simulink model "just_the_dynamics"  (R2017b)
settings: Solver=ode45  StartTime=0.0  StopTime=5000  RelTol=1e-3  EnableMultiTasking=on
undefined symbols (not defined in the file): a1, a2, a3, a4, b1, b2, b3, b4, c, c_mi_x, c_mi_y, c_mi_z, co_x, co_y, co_z, d, d_omega_R10, d_omega_R20, d_omega_R30, d_omega_R40, dfi_0, dpsi_0, dtheta_0, dx_0, dy_0, dz_0, f, fi_0, g, ga, h, Ixx, Iyy, Izz, Jr, K, L, m, psi_0, stateref, Tau, theta_0, V1_WP, V2_WP, V3_WP, V4_WP, x_0, y_0, z_0
settings Model: Creator=Jake  LastModifiedBy=Padraig Lysandrou
settings DataIOCC: LimitDataPoints=on  SaveFormat=Array  SignalLoggingSaveFormat=ModelDataLogs
settings OptimizationCC: InitFltsAndDblsToZero=on  LifeSpan=inf
settings DebuggingCC: SaveWithParameterizedLinksMsg=none  UnderspecifiedInitializationDetection=Classic  MergeDetectMultiDrivingBlocksExec=none  SignalResolutionControl=TryResolveAllWithWarning  SolverPrmCheckMsg=warning  MultiTaskDSMMsg=warning  MultiTaskCondExecSysMsg=none  FcnCallInpInsideContextMsg=warning  StrictBusMsg=Warning  SFUnexpectedBacktrackingDiag=warning  SFNoUnconditionalDefaultTransitionDiag=warning  SFExecutionAtInitializationDiag=none
settings HardwareCC: ProdBitPerPointer=32  ProdBitPerSizeT=32  ProdBitPerPtrDiffT=32  ProdLargestAtomicFloat=None  ProdIntDivRoundTo=Undefined  ProdEndianess=Unspecified  ProdWordSize=32  ProdHWDeviceType=32-bit Generic
settings ModelReferenceCC: PropagateSignalLabelsOutOfModel=off
settings SFSimCC: SimParseCustomCode=off
settings CodeAppCC: StateflowObjectComments=on
settings GRTTargetCC: TargetFcnLib=ansi_tfl_tmw.mat  TargetLangStandard=C89/C90 (ANSI)  CombineOutputUpdateFcns=off  GRTInterface=on
settings ConfigComp: CovMetricSettings=dw  CovHtmlReporting=on  CovSaveCumulativeToWorkspaceVar=on  CovSaveSingleToWorkspaceVar=on  CovExternalEMLEnable=off

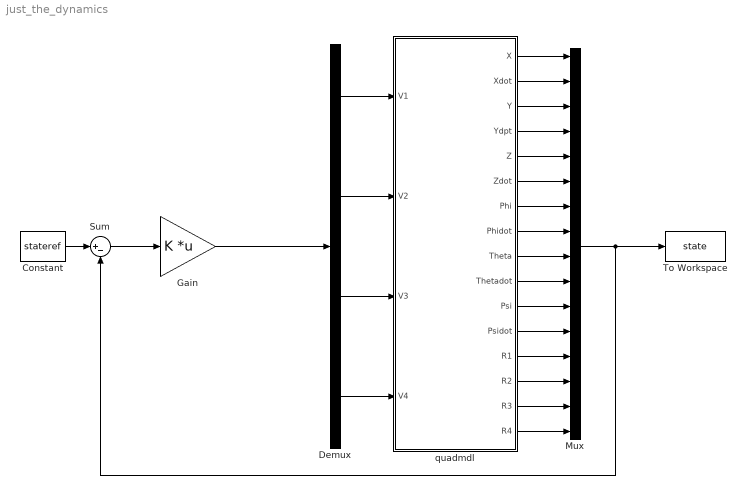
== system just_the_dynamics ==
  Constant : Constant  Value=stateref
  Demux : Demux
  Gain : Gain  Gain=K  Multiplication=Matrix(K*u) (u vector)
  Mux : Mux  Inputs=16
  Sum : Sum  Inputs=|+-
  To Workspace : ToWorkspace  VariableName=state  SaveFormat=Timeseries  SampleTime=-1
  quadmdl : Subsystem
  wires:
  quadmdl/1(X) -> Mux/1
  quadmdl/2(Xdot) -> Mux/2
  quadmdl/3(Y) -> Mux/3
  quadmdl/4(Ydpt) -> Mux/4
  quadmdl/5(Z) -> Mux/5
  quadmdl/6(Zdot) -> Mux/6
  quadmdl/7(Phi) -> Mux/7
  quadmdl/8(Phidot) -> Mux/8
  quadmdl/9(Theta) -> Mux/9
  quadmdl/10(Thetadot) -> Mux/10
  quadmdl/11(Psi) -> Mux/11
  quadmdl/12(Psidot) -> Mux/12
  quadmdl/13(R1) -> Mux/13
  quadmdl/14(R2) -> Mux/14
  quadmdl/15(R3) -> Mux/15
  quadmdl/16(R4) -> Mux/16
  Demux/1 -> quadmdl/1(V1)
  Demux/2 -> quadmdl/2(V2)
  Demux/3 -> quadmdl/3(V3)
  Demux/4 -> quadmdl/4(V4)
  Mux/1 -> Sum/2, To Workspace/1
  Gain/1 -> Demux/1
  Sum/1 -> Gain/1
  Constant/1 -> Sum/1

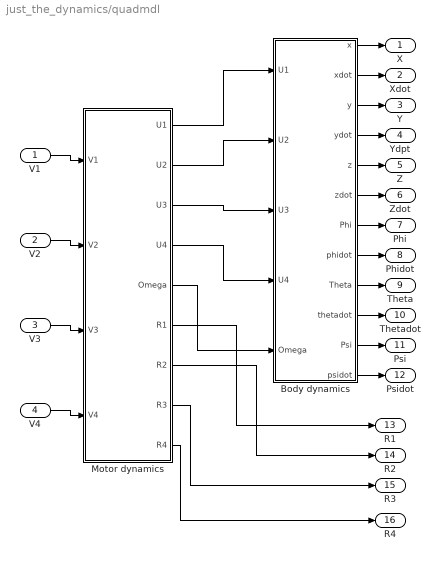
== system just_the_dynamics/quadmdl ==
  V1 : Inport
  V2 : Inport  Port=2
  V3 : Inport  Port=3
  V4 : Inport  Port=4
  Body dynamics : Subsystem
  Motor dynamics : Subsystem
  X : Outport
  Xdot : Outport  Port=2
  Y : Outport  Port=3
  Ydpt : Outport  Port=4
  Z : Outport  Port=5
  Zdot : Outport  Port=6
  Phi : Outport  Port=7
  Phidot : Outport  Port=8
  Theta : Outport  Port=9
  Thetadot : Outport  Port=10
  Psi : Outport  Port=11
  Psidot : Outport  Port=12
  R1 : Outport  Port=13
  R2 : Outport  Port=14
  R3 : Outport  Port=15
  R4 : Outport  Port=16
  wires:
  Motor dynamics/1(U1) -> Body dynamics/1(U1)
  Motor dynamics/2(U2) -> Body dynamics/2(U2)
  Motor dynamics/3(U3) -> Body dynamics/3(U3)
  Motor dynamics/4(U4) -> Body dynamics/4(U4)
  Motor dynamics/5(Omega) -> Body dynamics/5(Omega)
  Body dynamics/7(Phi) -> Phi/1
  Body dynamics/9(Theta) -> Theta/1
  Body dynamics/11(Psi) -> Psi/1
  Body dynamics/1(x) -> X/1
  V1/1 -> Motor dynamics/1(V1)
  Body dynamics/3(y) -> Y/1
  V2/1 -> Motor dynamics/2(V2)
  Body dynamics/5(z) -> Z/1
  V3/1 -> Motor dynamics/3(V3)
  V4/1 -> Motor dynamics/4(V4)
  Body dynamics/2(xdot) -> Xdot/1
  Body dynamics/4(ydot) -> Ydpt/1
  Body dynamics/6(zdot) -> Zdot/1
  Body dynamics/8(phidot) -> Phidot/1
  Body dynamics/10(thetadot) -> Thetadot/1
  Body dynamics/12(psidot) -> Psidot/1
  Motor dynamics/6(R1) -> R1/1
  Motor dynamics/7(R2) -> R2/1
  Motor dynamics/8(R3) -> R3/1
  Motor dynamics/9(R4) -> R4/1

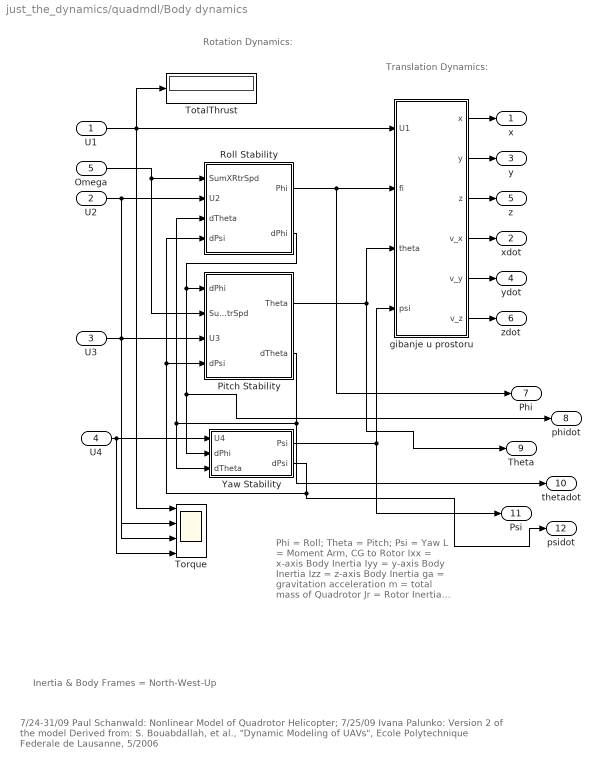
== system just_the_dynamics/quadmdl/Body dynamics ==
  note: Inertia & Body Frames = North-West-Up
  note: Rotation
      | Dynamics:
  note: Translation
      | Dynamics:
  note: Phi = Roll; Theta = Pitch; Psi = Yaw
      | L = Moment Arm, CG to Rotor
      | Ixx = x-axis Body Inertia
      | Iyy = y-axis Body Inertia
      | Izz = z-axis Body Inertia
      | ga = gravitation acceleration
      | m = total mass of Quadrotor
      | Jr = Rotor Inertia
      | a,b = Volts-to-Rotor Speed Consts
      | c,d,e = RtrSpd-to-Thrust Fcn Consts
      | f,g,h = RtrSpd-to-Drag Fcn Consts
      | Tau = Motor Time Const
  note: 7/24-31/09  Paul Schanwald:  Nonlinear Model of Quadrotor Helicopter; 7/25/09 Ivana Palunko: Version 2 of the model
      | Derived from: S. Bouabdallah, et al., "Dynamic Modeling of UAVs", Ecole Polytechnique Federale de Lausanne, 5/2006
  U1 : Inport
  U2 : Inport  Port=2
  U3 : Inport  Port=3
  U4 : Inport  Port=4
  Omega : Inport  Port=5
  Pitch Stability : Subsystem
  Roll Stability : Subsystem
  Torque : Scope  NumInputPorts=4
  TotalThrust : Display
  Yaw Stability : Subsystem
  gibanje u prostoru : Subsystem
  x : Outport
  xdot : Outport  Port=2
  y : Outport  Port=3
  ydot : Outport  Port=4
  z : Outport  Port=5
  zdot : Outport  Port=6
  Phi : Outport  Port=7
  phidot : Outport  Port=8
  Theta : Outport  Port=9
  thetadot : Outport  Port=10
  Psi : Outport  Port=11
  psidot : Outport  Port=12
  wires:
  U4/1 -> Yaw Stability/1(U4), Torque/4
  U3/1 -> Pitch Stability/3(U3), Torque/3
  U1/1 -> TotalThrust/1, gibanje u prostoru/1(U1), Torque/1
  gibanje u prostoru/3(z) -> z/1
  gibanje u prostoru/2(y) -> y/1
  gibanje u prostoru/1(x) -> x/1
  U2/1 -> Roll Stability/2(U2), Torque/2
  Omega/1 -> Roll Stability/1(SumXRtrSpd), Pitch Stability/2(SumYRtrSpd)
  Roll Stability/2(dPhi) -> Pitch Stability/1(dPhi), phidot/1, Yaw Stability/2(dPhi)
  Pitch Stability/2(dTheta) -> thetadot/1, Yaw Stability/3(dTheta), Roll Stability/3(dTheta)
  Yaw Stability/2(dPsi) -> psidot/1, Roll Stability/4(dPsi), Pitch Stability/4(dPsi)
  Roll Stability/1(Phi) -> gibanje u prostoru/2(fi), Phi/1
  Pitch Stability/1(Theta) -> gibanje u prostoru/3(theta), Theta/1
  Yaw Stability/1(Psi) -> Psi/1, gibanje u prostoru/4(psi)
  gibanje u prostoru/6(v_z) -> zdot/1
  gibanje u prostoru/4(v_x) -> xdot/1
  gibanje u prostoru/5(v_y) -> ydot/1

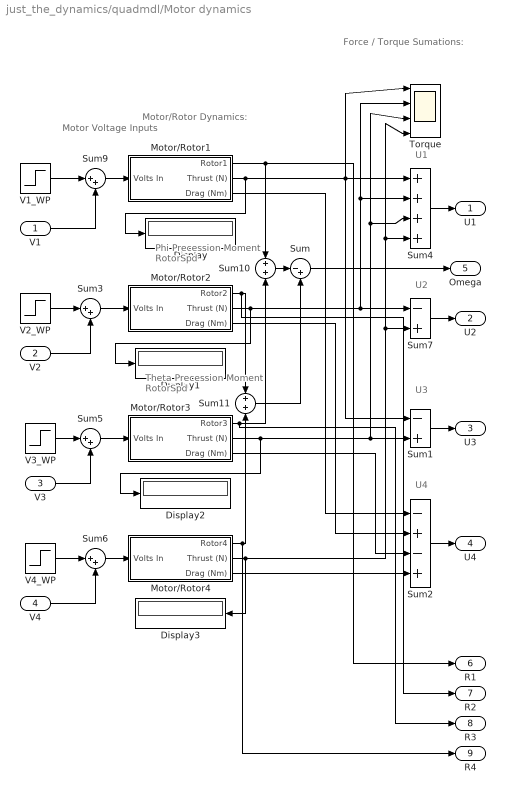
== system just_the_dynamics/quadmdl/Motor dynamics ==
  note: Theta Precession
      | Moment RotorSpd
  note: Phi Precession
      | Moment RotorSpd
  note: Motor/Rotor
      | Dynamics:
  note: Force / Torque
      | Sumations:
  note: Motor
      | Voltage
      | Inputs
  note: U4
  note: U3
  note: U2
  note: U1
  V1 : Inport
  V2 : Inport  Port=2
  V3 : Inport  Port=3
  V4 : Inport  Port=4
  Display{,1..3} (4 alike) : Display
  Motor/Rotor1 : Subsystem
  Motor/Rotor2 : Subsystem
  Motor/Rotor3 : Subsystem
  Motor/Rotor4 : Subsystem
  Sum : Sum  Inputs=|-+
  Sum1 : Sum  Inputs=-+
  Sum10 : Sum  Inputs=+|+
  Sum11 : Sum  Inputs=+|+
  Sum2 : Sum  Inputs=-+-+
  Sum{3,5..6,9} (4 alike) : Sum  Inputs=|++
  Sum4 : Sum  Inputs=++++
  Sum7 : Sum  Inputs=-+
  Torque : Scope  NumInputPorts=4
  V1_WP : Step  Time=0  Before=V1_WP  After=V1_WP  SampleTime=0
  V2_WP : Step  Time=0  Before=V2_WP  After=V2_WP  SampleTime=0
  V3_WP : Step  Time=0  Before=V3_WP  After=V3_WP  SampleTime=0
  V4_WP : Step  Time=0  Before=V4_WP  After=V4_WP  SampleTime=0
  U1 : Outport
  U2 : Outport  Port=2
  U3 : Outport  Port=3
  U4 : Outport  Port=4
  Omega : Outport  Port=5
  R1 : Outport  Port=6
  R2 : Outport  Port=7
  R3 : Outport  Port=8
  R4 : Outport  Port=9
  wires:
  Sum11/1 -> Sum/2
  Sum10/1 -> Sum/1
  Motor/Rotor4/1(Rotor4) -> R4/1, Sum11/2
  Motor/Rotor4/2(Thrust (N)) -> Display3/1, Torque/4, Sum4/4, Sum7/2
  Motor/Rotor4/3(Drag (Nm)) -> Sum2/4
  Motor/Rotor3/3(Drag (Nm)) -> Sum2/3
  Motor/Rotor3/1(Rotor3) -> R3/1, Sum10/2
  Motor/Rotor3/2(Thrust (N)) -> Display2/1, Torque/3, Sum4/3, Sum1/2
  Motor/Rotor2/1(Rotor2) -> R2/1, Sum11/1
  Motor/Rotor2/3(Drag (Nm)) -> Sum2/2
  Motor/Rotor2/2(Thrust (N)) -> Display1/1, Torque/2, Sum4/2, Sum7/1
  Motor/Rotor1/1(Rotor1) -> R1/1, Sum10/1
  Motor/Rotor1/3(Drag (Nm)) -> Sum2/1
  Motor/Rotor1/2(Thrust (N)) -> Display/1, Sum4/1, Torque/1, Sum1/1
  Sum4/1 -> U1/1
  Sum/1 -> Omega/1
  Sum7/1 -> U2/1
  Sum1/1 -> U3/1
  Sum2/1 -> U4/1
  Sum9/1 -> Motor/Rotor1/1(Volts In)
  V1_WP/1 -> Sum9/1
  V2_WP/1 -> Sum3/1
  Sum3/1 -> Motor/Rotor2/1(Volts In)
  V3_WP/1 -> Sum5/1
  Sum5/1 -> Motor/Rotor3/1(Volts In)
  V4_WP/1 -> Sum6/1
  Sum6/1 -> Motor/Rotor4/1(Volts In)
  V1/1 -> Sum9/2
  V2/1 -> Sum3/2
  V3/1 -> Sum5/2
  V4/1 -> Sum6/2

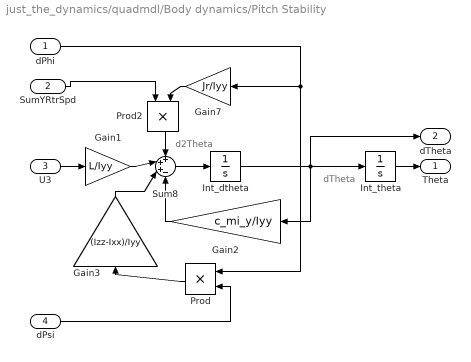
== system just_the_dynamics/quadmdl/Body dynamics/Pitch Stability ==
  note: d2Theta
  note: dTheta
  dPhi : Inport
  SumYRtrSpd : Inport  Port=2
  U3 : Inport  Port=3
  dPsi : Inport  Port=4
  Gain1 : Gain  Gain=L/Iyy
  Gain2 : Gain  Gain=c_mi_y/Iyy
  Gain3 : Gain  Gain=(Izz-Ixx)/Iyy
  Gain7 : Gain  Gain=Jr/Iyy
  Int_dtheta : Integrator  InitialCondition=dtheta_0
  Int_theta : Integrator  InitialCondition=theta_0  UpperSaturationLimit=pi/2  LowerSaturationLimit=-pi/2
  Prod : Product  RndMeth=Zero
  Prod2 : Product  RndMeth=Zero
  Sum8 : Sum  Inputs=+++-
  Theta : Outport
  dTheta : Outport  Port=2
  wires:
  Gain2/1 -> Sum8/4
  dPhi/1 -> Prod/1, Gain7/1
  Int_theta/1 -> Theta/1
  U3/1 -> Gain1/1
  SumYRtrSpd/1 -> Prod2/1
  dPsi/1 -> Prod/2
  Int_dtheta/1 -> dTheta/1, Int_theta/1, Gain2/1
  Sum8/1 -> Int_dtheta/1
  Gain1/1 -> Sum8/2
  Gain7/1 -> Prod2/2
  Gain3/1 -> Sum8/3
  Prod/1 -> Gain3/1
  Prod2/1 -> Sum8/1

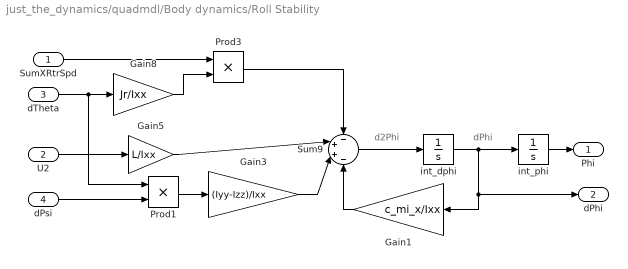
== system just_the_dynamics/quadmdl/Body dynamics/Roll Stability ==
  note: d2Phi
  note: dPhi
  SumXRtrSpd : Inport
  U2 : Inport  Port=2
  dTheta : Inport  Port=3
  dPsi : Inport  Port=4
  Gain1 : Gain  Gain=c_mi_x/Ixx
  Gain3 : Gain  Gain=(Iyy-Izz)/Ixx
  Gain5 : Gain  Gain=L/Ixx
  Gain8 : Gain  Gain=Jr/Ixx
  Prod1 : Product  RndMeth=Zero
  Prod3 : Product  RndMeth=Zero
  Sum9 : Sum  Inputs=-++-
  int_dphi : Integrator  InitialCondition=dfi_0
  int_phi : Integrator  InitialCondition=fi_0  UpperSaturationLimit=pi/2  LowerSaturationLimit=-pi/2
  Phi : Outport
  dPhi : Outport  Port=2
  wires:
  dPsi/1 -> Prod1/2
  dTheta/1 -> Prod1/1, Gain8/1
  Prod3/1 -> Sum9/1
  SumXRtrSpd/1 -> Prod3/1
  Gain8/1 -> Prod3/2
  int_phi/1 -> Phi/1
  U2/1 -> Gain5/1
  int_dphi/1 -> Gain1/1, dPhi/1, int_phi/1
  Sum9/1 -> int_dphi/1
  Gain5/1 -> Sum9/2
  Gain1/1 -> Sum9/4
  Gain3/1 -> Sum9/3
  Prod1/1 -> Gain3/1

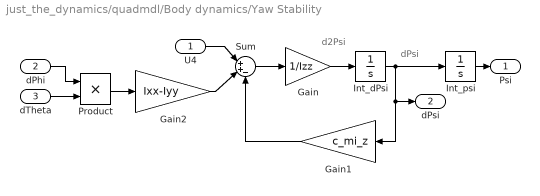
== system just_the_dynamics/quadmdl/Body dynamics/Yaw Stability ==
  note: dPsi
  note: d2Psi
  U4 : Inport
  dPhi : Inport  Port=2
  dTheta : Inport  Port=3
  Gain : Gain  Gain=1/Izz
  Gain1 : Gain  Gain=c_mi_z
  Gain2 : Gain  Gain=Ixx-Iyy
  Int_dPsi : Integrator  InitialCondition=dpsi_0
  Int_psi : Integrator  InitialCondition=psi_0
  Product : Product  RndMeth=Zero
  Sum : Sum  Inputs=|++-
  Psi : Outport
  dPsi : Outport  Port=2
  wires:
  Sum/1 -> Gain/1
  U4/1 -> Sum/1
  Int_psi/1 -> Psi/1
  Gain/1 -> Int_dPsi/1
  Int_dPsi/1 -> Gain1/1, dPsi/1, Int_psi/1
  Gain1/1 -> Sum/3
  Gain2/1 -> Sum/2
  dPhi/1 -> Product/1
  dTheta/1 -> Product/2
  Product/1 -> Gain2/1

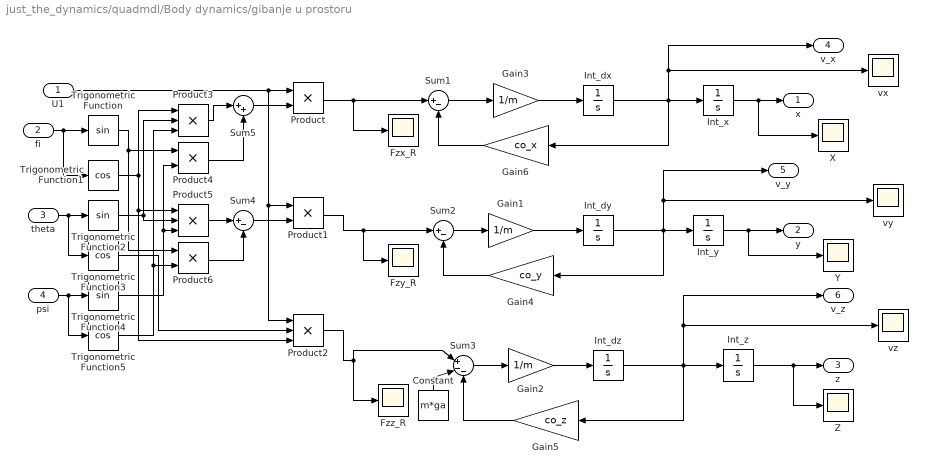
== system just_the_dynamics/quadmdl/Body dynamics/gibanje u prostoru ==
  U1 : Inport
  fi : Inport  Port=2
  theta : Inport  Port=3
  psi : Inport  Port=4
  Constant : Constant  Value=m*ga
  Fzx_R : Scope
  Fzy_R : Scope
  Fzz_R : Scope
  Gain1 : Gain  Gain=1/m
  Gain2 : Gain  Gain=1/m
  Gain3 : Gain  Gain=1/m
  Gain4 : Gain  Gain=co_y
  Gain5 : Gain  Gain=co_z
  Gain6 : Gain  Gain=co_x
  Int_dx : Integrator  InitialCondition=dx_0  LimitOutput=on  UpperSaturationLimit=10  LowerSaturationLimit=-10
  Int_dy : Integrator  InitialCondition=dy_0  LimitOutput=on  UpperSaturationLimit=10  LowerSaturationLimit=-10
  Int_dz : Integrator  InitialCondition=dz_0  LimitOutput=on  UpperSaturationLimit=10  LowerSaturationLimit=-10
  Int_x : Integrator  InitialCondition=x_0
  Int_y : Integrator  InitialCondition=y_0
  Int_z : Integrator  InitialCondition=z_0
  Product{,1,4,6} (4 alike) : Product  RndMeth=Zero
  Product2 : Product  Inputs=3  RndMeth=Zero
  Product3 : Product  Inputs=3  RndMeth=Zero
  Product5 : Product  Inputs=3  RndMeth=Zero
  Sum1 : Sum  Inputs=|+-
  Sum2 : Sum  Inputs=|+-
  Sum3 : Sum  Inputs=|+--
  Sum4 : Sum  Inputs=|+-
  Sum5 : Sum  Inputs=|++
  Trigonometric Function : Trigonometry
  Trigonometric Function1 : Trigonometry  Operator=cos
  Trigonometric Function2 : Trigonometry
  Trigonometric Function3 : Trigonometry  Operator=cos
  Trigonometric Function4 : Trigonometry
  Trigonometric Function5 : Trigonometry  Operator=cos
  X : Scope
  Y : Scope
  Z : Scope
  vx : Scope
  vy : Scope
  vz : Scope
  x : Outport
  y : Outport  Port=2
  z : Outport  Port=3
  v_x : Outport  Port=4
  v_y : Outport  Port=5
  v_z : Outport  Port=6
  wires:
  Gain5/1 -> Sum3/3
  Constant/1 -> Sum3/2
  Gain4/1 -> Sum2/2
  Sum3/1 -> Gain2/1
  Gain6/1 -> Sum1/2
  Product2/1 -> Sum3/1, Fzz_R/1
  Sum2/1 -> Gain1/1
  Product1/1 -> Fzy_R/1, Sum2/1
  Gain2/1 -> Int_dz/1
  Sum1/1 -> Gain3/1
  Product/1 -> Fzx_R/1, Sum1/1
  U1/1 -> Product/1, Product1/1, Product2/1
  Int_y/1 -> Y/1, y/1
  Int_x/1 -> X/1, x/1
  Int_z/1 -> Z/1, z/1
  Int_dx/1 -> Gain6/1, vx/1, v_x/1, Int_x/1
  Int_dy/1 -> Gain4/1, Int_y/1, vy/1, v_y/1
  Int_dz/1 -> vz/1, v_z/1, Gain5/1, Int_z/1
  Gain1/1 -> Int_dy/1
  Gain3/1 -> Int_dx/1
  Sum4/1 -> Product1/2
  Sum5/1 -> Product/2
  Product3/1 -> Sum5/1
  Product4/1 -> Sum5/2
  Product5/1 -> Sum4/1
  Product6/1 -> Sum4/2
  psi/1 -> Trigonometric Function4/1, Trigonometric Function5/1
  theta/1 -> Trigonometric Function2/1, Trigonometric Function3/1
  fi/1 -> Trigonometric Function/1, Trigonometric Function1/1
  Trigonometric Function/1 -> Product4/1, Product6/1
  Trigonometric Function1/1 -> Product3/1, Product5/1, Product2/3
  Trigonometric Function2/1 -> Product3/2, Product5/2
  Trigonometric Function5/1 -> Product3/3, Product6/2
  Trigonometric Function4/1 -> Product4/2, Product5/3
  Trigonometric Function3/1 -> Product2/2

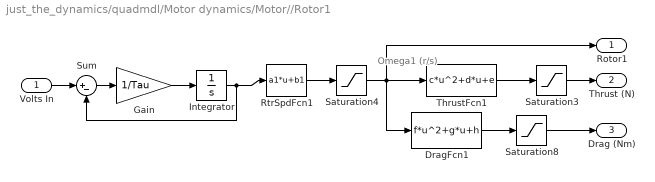
== system just_the_dynamics/quadmdl/Motor dynamics/Motor//Rotor1 ==
  note: Omega1
      | (r/s)
  Volts In : Inport
  DragFcn1 : Fcn  Expr=f*u^2+g*u+h
  Gain : Gain  Gain=1/Tau
  Integrator : Integrator  InitialCondition=d_omega_R10
  RtrSpdFcn1 : Fcn  Expr=a1*u+b1
  Saturation3 : Saturate  UpperLimit=15  LowerLimit=0
  Saturation4 : Saturate  UpperLimit=250  LowerLimit=0
  Saturation8 : Saturate  UpperLimit=1  LowerLimit=0
  Sum : Sum  Inputs=|+-
  ThrustFcn1 : Fcn  Expr=c*u^2+d*u+e
  Rotor1 : Outport
  Thrust (N) : Outport  Port=2
  Drag (Nm) : Outport  Port=3
  wires:
  Volts In/1 -> Sum/1
  Sum/1 -> Gain/1
  Integrator/1 -> RtrSpdFcn1/1, Sum/2
  Gain/1 -> Integrator/1
  Saturation3/1 -> Thrust (N)/1
  Saturation8/1 -> Drag (Nm)/1
  DragFcn1/1 -> Saturation8/1
  Saturation4/1 -> Rotor1/1, DragFcn1/1, ThrustFcn1/1
  RtrSpdFcn1/1 -> Saturation4/1
  ThrustFcn1/1 -> Saturation3/1

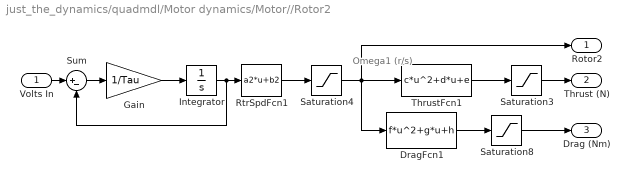
== system just_the_dynamics/quadmdl/Motor dynamics/Motor//Rotor2 ==
  note: Omega1
      | (r/s)
  Volts In : Inport
  DragFcn1 : Fcn  Expr=f*u^2+g*u+h
  Gain : Gain  Gain=1/Tau
  Integrator : Integrator  InitialCondition=d_omega_R20
  RtrSpdFcn1 : Fcn  Expr=a2*u+b2
  Saturation3 : Saturate  UpperLimit=15  LowerLimit=0
  Saturation4 : Saturate  UpperLimit=250  LowerLimit=0
  Saturation8 : Saturate  UpperLimit=1  LowerLimit=0
  Sum : Sum  Inputs=|+-
  ThrustFcn1 : Fcn  Expr=c*u^2+d*u+e
  Rotor2 : Outport
  Thrust (N) : Outport  Port=2
  Drag (Nm) : Outport  Port=3
  wires:
  Volts In/1 -> Sum/1
  Sum/1 -> Gain/1
  Integrator/1 -> RtrSpdFcn1/1, Sum/2
  Gain/1 -> Integrator/1
  Saturation3/1 -> Thrust (N)/1
  Saturation8/1 -> Drag (Nm)/1
  DragFcn1/1 -> Saturation8/1
  ThrustFcn1/1 -> Saturation3/1
  Saturation4/1 -> Rotor2/1, DragFcn1/1, ThrustFcn1/1
  RtrSpdFcn1/1 -> Saturation4/1

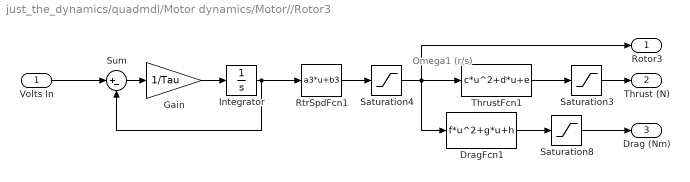
== system just_the_dynamics/quadmdl/Motor dynamics/Motor//Rotor3 ==
  note: Omega1
      | (r/s)
  Volts In : Inport
  DragFcn1 : Fcn  Expr=f*u^2+g*u+h
  Gain : Gain  Gain=1/Tau
  Integrator : Integrator  InitialCondition=d_omega_R30
  RtrSpdFcn1 : Fcn  Expr=a3*u+b3
  Saturation3 : Saturate  UpperLimit=15  LowerLimit=0
  Saturation4 : Saturate  UpperLimit=250  LowerLimit=0
  Saturation8 : Saturate  UpperLimit=1  LowerLimit=0
  Sum : Sum  Inputs=|+-
  ThrustFcn1 : Fcn  Expr=c*u^2+d*u+e
  Rotor3 : Outport
  Thrust (N) : Outport  Port=2
  Drag (Nm) : Outport  Port=3
  wires:
  Volts In/1 -> Sum/1
  Sum/1 -> Gain/1
  Integrator/1 -> RtrSpdFcn1/1, Sum/2
  Gain/1 -> Integrator/1
  Saturation3/1 -> Thrust (N)/1
  Saturation8/1 -> Drag (Nm)/1
  DragFcn1/1 -> Saturation8/1
  ThrustFcn1/1 -> Saturation3/1
  Saturation4/1 -> Rotor3/1, DragFcn1/1, ThrustFcn1/1
  RtrSpdFcn1/1 -> Saturation4/1

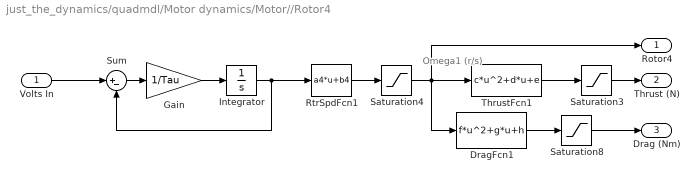
== system just_the_dynamics/quadmdl/Motor dynamics/Motor//Rotor4 ==
  note: Omega1
      | (r/s)
  Volts In : Inport
  DragFcn1 : Fcn  Expr=f*u^2+g*u+h
  Gain : Gain  Gain=1/Tau
  Integrator : Integrator  InitialCondition=d_omega_R40
  RtrSpdFcn1 : Fcn  Expr=a4*u+b4
  Saturation3 : Saturate  UpperLimit=15  LowerLimit=0
  Saturation4 : Saturate  UpperLimit=250  LowerLimit=0
  Saturation8 : Saturate  UpperLimit=1  LowerLimit=0
  Sum : Sum  Inputs=|+-
  ThrustFcn1 : Fcn  Expr=c*u^2+d*u+e
  Rotor4 : Outport
  Thrust (N) : Outport  Port=2
  Drag (Nm) : Outport  Port=3
  wires:
  Volts In/1 -> Sum/1
  Sum/1 -> Gain/1
  Integrator/1 -> RtrSpdFcn1/1, Sum/2
  Gain/1 -> Integrator/1
  Saturation3/1 -> Thrust (N)/1
  Saturation8/1 -> Drag (Nm)/1
  DragFcn1/1 -> Saturation8/1
  ThrustFcn1/1 -> Saturation3/1
  Saturation4/1 -> Rotor4/1, DragFcn1/1, ThrustFcn1/1
  RtrSpdFcn1/1 -> Saturation4/1
